simulink model "VendingMachine"  (R2020b)
settings: Solver=VariableStepAuto  StartTime=0.0  StopTime=100  RelTol=1e-3
settings Model: Creator=BIDITA PAUL  LastModifiedBy=BIDITA PAUL

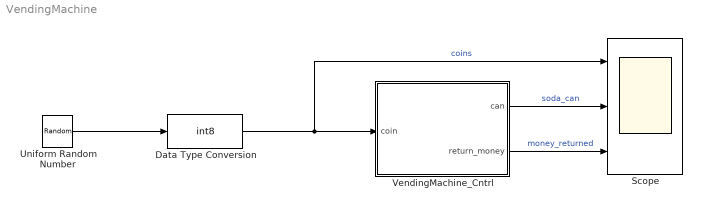
== system VendingMachine ==
  Data Type Conversion : DataTypeConversion  OutDataTypeStr=int8  RndMeth=Nearest  SaturateOnIntegerOverflow=on
  Scope : Scope  NumInputPorts=3
  Uniform Random Number : UniformRandomNumber  Minimum=0  Maximum=2  SampleTime=1
  VendingMachine_Cntrl : Stateflow chart  TreatAsAtomicUnit=on
  wires:
  Data Type Conversion/1 -> Scope/1, VendingMachine_Cntrl/1(coin)  "coins"
  VendingMachine_Cntrl/1(can) -> Scope/2  "soda_can"
  VendingMachine_Cntrl/2(return_money) -> Scope/3  "money_returned"
  Uniform Random Number/1 -> Data Type Conversion/1

== stateflow chart VendingMachine/VendingMachine_Cntrl ==
  state S0
    entry:
    return_money = 0;
  state S10
  state S5
  state S20
  state S15
  state S30
  state S25
  S25 -> S0 : {return_money=0; can=0;}
  (default) -> S0
  S30 -> S0 : {return_money = 5; can = 0;}
  S0 -> S5 [order 2] : [coin==1]{can =0;}
  S0 -> S10 [order 1] : [coin==2]{can=0;}
  S5 -> S10 [order 2] : [coin==1]{can=0;}
  S10 -> S15 [order 2] : [coin==1]{can=0;}
  S10 -> S20 [order 1] : [coin==2]{can=0;}
  S5 -> S15 [order 1] : [coin==2]{can=0;}
  S15 -> S20 [order 2] : [coin==1]{can=0;}
  S20 -> S30 [order 2] : [coin==2]{can =1;}
  S20 -> S25 [order 1] : [coin==1]{can=1;}
  S15 -> S25 [order 1] : [coin==2]{can=1;}
  data: coin input; can output; return_money output
